simulink subsystem "ConventionalVehicle"  (R2023b)
settings: Solver=VariableStepAuto  StartTime=0.0  StopTime=10.0  RelTol=1e-3
settings Model: Creator=The MathWorks, Inc.  LastModifiedBy=The MathWorks, Inc.

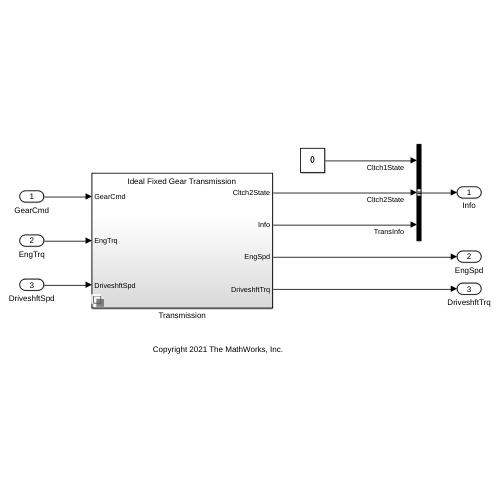
[thumbnail: Simulink's stored preview of the top-level diagram]
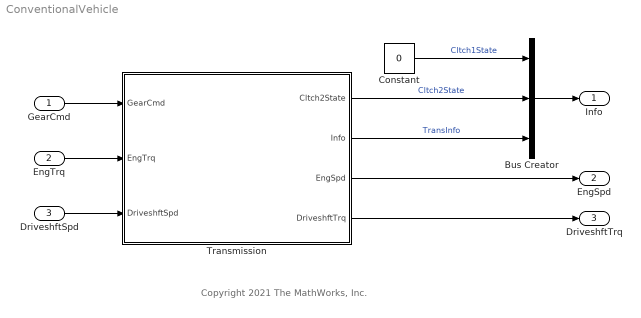
== system ConventionalVehicle ==
  note: Copyright 2021 The MathWorks, Inc.
  GearCmd : Inport
  EngTrq : Inport  Port=2
  DriveshftSpd : Inport  Port=3
  Bus Creator : BusCreator  Inputs=3
  Constant : Constant  Value=0  SampleTime=-1
  Transmission : Subsystem  Variant=on  VariantControlMode=label  VariantControl=1  LabelModeActiveChoice=Ideal Fixed Gear Transmission
  Info : Outport
  EngSpd : Outport  Port=2
  DriveshftTrq : Outport  Port=3
  wires:
  Constant/1 -> Bus Creator/1  "Cltch1State"
  Transmission/2(Info) -> Bus Creator/3  "TransInfo"
  EngTrq/1 -> Transmission/2(EngTrq)
  Transmission/1(Cltch2State) -> Bus Creator/2  "Cltch2State"
  GearCmd/1 -> Transmission/1(GearCmd)
  DriveshftSpd/1 -> Transmission/3(DriveshftSpd)
  Bus Creator/1 -> Info/1
  Transmission/4(DriveshftTrq) -> DriveshftTrq/1
  Transmission/3(EngSpd) -> EngSpd/1

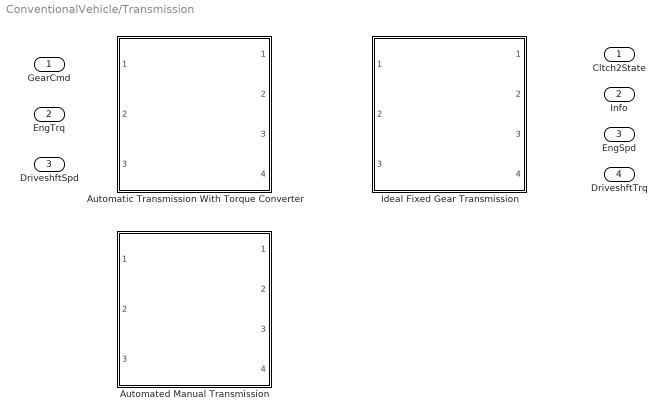
== system ConventionalVehicle/Transmission ==
  GearCmd : Inport
  EngTrq : Inport  Port=2
  DriveshftSpd : Inport  Port=3
  Automated Manual Transmission : Subsystem  VariantControl=Automated Manual Transmission  ReferencedSubsystem=AutomatedManualTransmission
  Automatic Transmission With Torque Converter : Subsystem  VariantControl=Automatic Transmission With Torque Converter  ReferencedSubsystem=AutomaticTransmissionWithTorqueConverter
  Ideal Fixed Gear Transmission : Subsystem  VariantControl=Ideal Fixed Gear Transmission  ReferencedSubsystem=IdealFixedGearTransmission
  Cltch2State : Outport
  Info : Outport  Port=2
  EngSpd : Outport  Port=3
  DriveshftTrq : Outport  Port=4
